simulink model "Part1"  (R2018b)
settings: Solver=VariableStepAuto  StartTime=0.0  StopTime=10.0  RelTol=1e-3
settings Model: Creator=Rasouli  LastModifiedBy=Rasouli

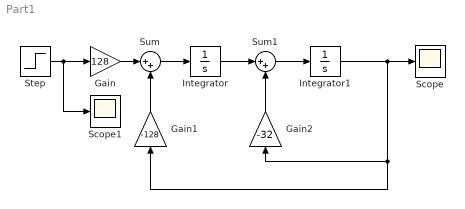
== system Part1 ==
  Gain : Gain  Gain=128
  Gain1 : Gain  Gain=-128
  Gain2 : Gain  Gain=-32
  Integrator : Integrator
  Integrator1 : Integrator
  Scope : Scope
  Scope1 : Scope
  Step : Step  Time=0.01  SampleTime=0
  Sum : Sum  Inputs=|++
  Sum1 : Sum  Inputs=|++
  wires:
  Sum/1 -> Integrator/1
  Step/1 -> Scope1/1, Gain/1
  Gain/1 -> Sum/1
  Gain2/1 -> Sum1/2
  Gain1/1 -> Sum/2
  Sum1/1 -> Integrator1/1
  Integrator/1 -> Sum1/1
  Integrator1/1 -> Scope/1, Gain1/1, Gain2/1
